simulink model "smlnk_hw3"  (R2019b)
settings: Solver=VariableStepAuto  StartTime=0.0  StopTime=30.0  RelTol=1e-3
undefined symbols (not defined in the file): K, k_r, L, ol, x0
settings Model: Creator=maximemeurisse  LastModifiedBy=maximemeurisse

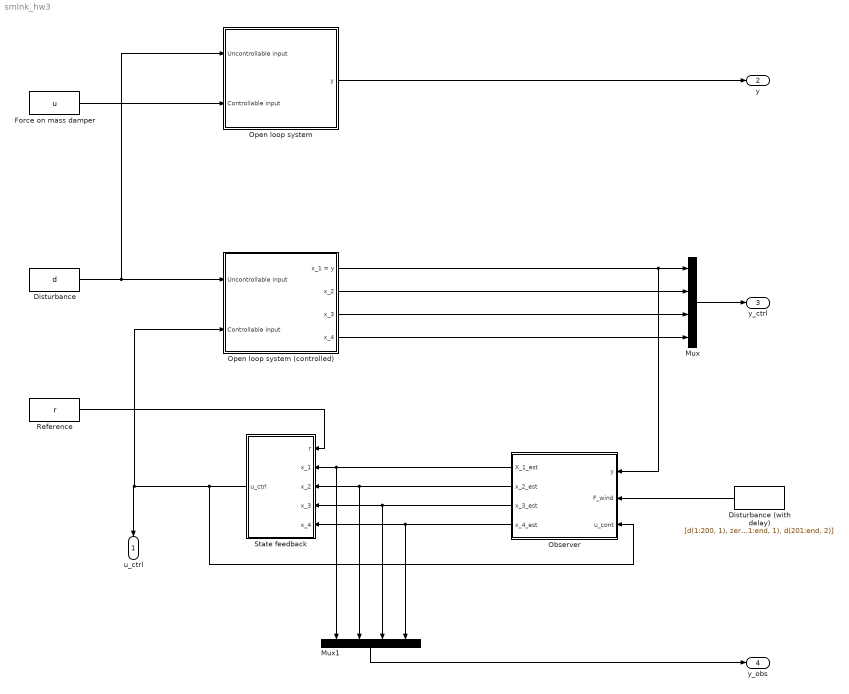
== system smlnk_hw3 ==
  Disturbance : FromWorkspace  VariableName=d  SampleTime=0
  Disturbance (with delay) : FromWorkspace  VariableName=[d(1:200, 1), zeros(200, 1); d(201:end, 1), d(201:end, 2)]  SampleTime=0
  Force on mass damper : FromWorkspace  VariableName=u  SampleTime=0
  Mux : Mux
  Mux1 : Mux
  Observer : Subsystem
  Open loop system : Subsystem
  Open loop system (controlled) : Subsystem
  Reference : FromWorkspace  VariableName=r  SampleTime=0
  State feedback : Subsystem
  u_ctrl : Outport
  y : Outport  Port=2
  y_ctrl : Outport  Port=3
  y_obs : Outport  Port=4
  wires:
  State feedback/1(u_ctrl) -> Observer/3(u_cont), Open loop system (controlled)/2(Controllable input), u_ctrl/1
  Observer/1(X_1_est) -> State feedback/2(x_1), Mux1/1
  Observer/2(x_2_est) -> State feedback/3(x_2), Mux1/2
  Reference/1 -> State feedback/1(r)
  Force on mass damper/1 -> Open loop system/2(Controllable input)
  Open loop system/1(y) -> y/1
  Mux/1 -> y_ctrl/1
  Mux1/1 -> y_obs/1
  Observer/3(x_3_est) -> State feedback/4(x_3), Mux1/3
  Observer/4(x_4_est) -> State feedback/5(x_4), Mux1/4
  Disturbance/1 -> Open loop system/1(Uncontrollable input), Open loop system (controlled)/1(Uncontrollable input)
  Open loop system (controlled)/2(x_2) -> Mux/2
  Open loop system (controlled)/3(x_3) -> Mux/3
  Open loop system (controlled)/4(x_4) -> Mux/4
  Open loop system (controlled)/1(x_1 = y) -> Observer/1(y), Mux/1
  Disturbance (with delay)/1 -> Observer/2(F_wind)

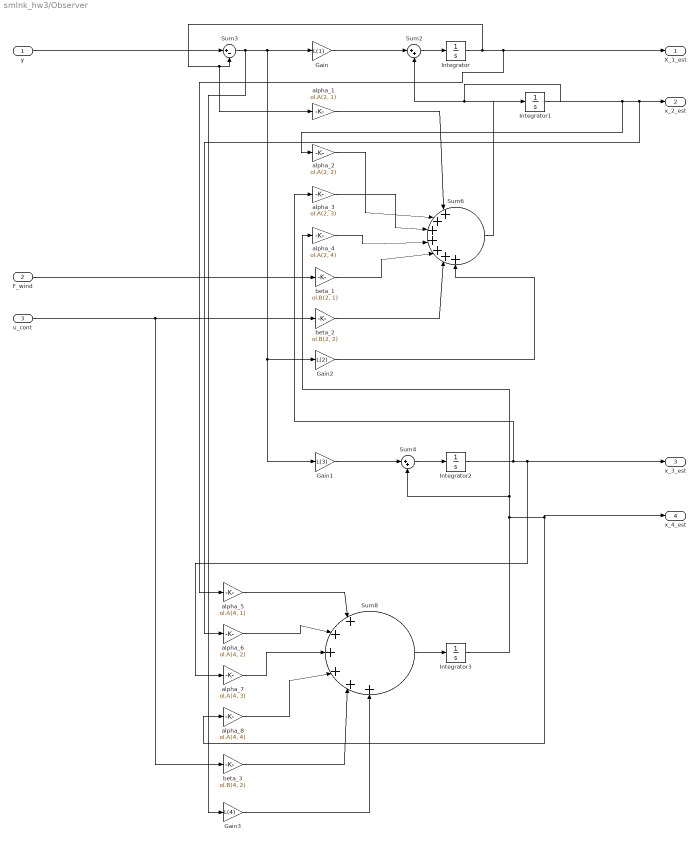
== system smlnk_hw3/Observer ==
  y : Inport
  F_wind : Inport  Port=2
  u_cont : Inport  Port=3
  Gain : Gain  Gain=L(1)
  Gain1 : Gain  Gain=L(3)
  Gain2 : Gain  Gain=L(2)
  Gain3 : Gain  Gain=L(4)
  Integrator{,1..3} (4 alike) : Integrator
  Sum2 : Sum  Inputs=|++
  Sum3 : Sum  Inputs=|+-
  Sum4 : Sum  Inputs=|++
  Sum6 : Sum  Inputs=|+++++++
  Sum8 : Sum  Inputs=|++++++
  alpha_1 : Gain  Gain=ol.A(2, 1)
  alpha_2 : Gain  Gain=ol.A(2, 2)
  alpha_3 : Gain  Gain=ol.A(2, 3)
  alpha_4 : Gain  Gain=ol.A(2, 4)
  alpha_5 : Gain  Gain=ol.A(4, 1)
  alpha_6 : Gain  Gain=ol.A(4, 2)
  alpha_7 : Gain  Gain=ol.A(4, 3)
  alpha_8 : Gain  Gain=ol.A(4, 4)
  beta_1 : Gain  Gain=ol.B(2, 1)
  beta_2 : Gain  Gain=ol.B(2, 2)
  beta_3 : Gain  Gain=ol.B(4, 2)
  X_1_est : Outport
  x_2_est : Outport  Port=2
  x_3_est : Outport  Port=3
  x_4_est : Outport  Port=4
  wires:
  Integrator2/1 -> alpha_3/1, alpha_7/1, x_3_est/1
  alpha_8/1 -> Sum8/4
  F_wind/1 -> beta_1/1
  Sum8/1 -> Integrator3/1
  alpha_2/1 -> Sum6/2
  beta_1/1 -> Sum6/5
  Sum4/1 -> Integrator2/1
  Integrator1/1 -> alpha_2/1, alpha_6/1, x_2_est/1, Sum2/2
  alpha_3/1 -> Sum6/3
  u_cont/1 -> beta_3/1, beta_2/1
  Gain1/1 -> Sum4/1
  alpha_4/1 -> Sum6/4
  Integrator/1 -> alpha_5/1, X_1_est/1, Sum3/2, alpha_1/1
  beta_3/1 -> Sum8/5
  Sum3/1 -> Gain3/1, Gain1/1, Gain2/1, Gain/1
  alpha_5/1 -> Sum8/1
  y/1 -> Sum3/1
  alpha_1/1 -> Sum6/1
  Sum2/1 -> Integrator/1
  alpha_6/1 -> Sum8/2
  beta_2/1 -> Sum6/6
  Sum6/1 -> Integrator1/1
  Gain2/1 -> Sum6/7
  Gain3/1 -> Sum8/6
  alpha_7/1 -> Sum8/3
  Gain/1 -> Sum2/1
  Integrator3/1 -> alpha_4/1, Sum4/2, alpha_8/1, x_4_est/1

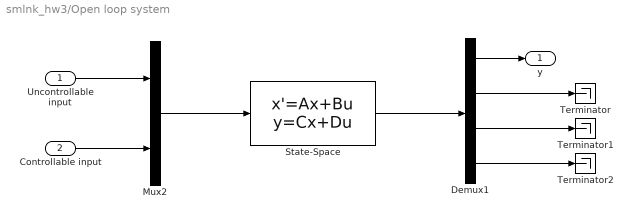
== system smlnk_hw3/Open loop system ==
  Uncontrollable input : Inport
  Controllable input : Inport  Port=2
  Demux1 : Demux
  Mux2 : Mux  Inputs=2
  State-Space : StateSpace  A=ol.A  B=ol.B  C=ol.C  D=ol.D  InitialCondition=x0
  Terminator : Terminator
  Terminator1 : Terminator
  Terminator2 : Terminator
  y : Outport
  wires:
  Controllable input/1 -> Mux2/2
  Uncontrollable input/1 -> Mux2/1
  Demux1/4 -> Terminator2/1
  Demux1/2 -> Terminator/1
  Demux1/3 -> Terminator1/1
  State-Space/1 -> Demux1/1
  Demux1/1 -> y/1
  Mux2/1 -> State-Space/1

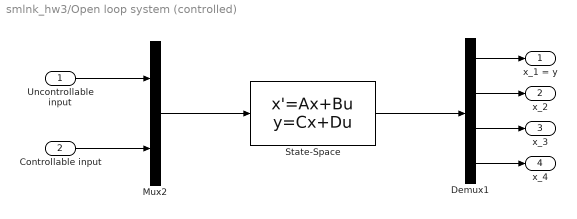
== system smlnk_hw3/Open loop system (controlled) ==
  Uncontrollable input : Inport
  Controllable input : Inport  Port=2
  Demux1 : Demux
  Mux2 : Mux  Inputs=2
  State-Space : StateSpace  A=ol.A  B=ol.B  C=ol.C  D=ol.D  InitialCondition=x0
  x_1 = y : Outport
  x_2 : Outport  Port=2
  x_3 : Outport  Port=3
  x_4 : Outport  Port=4
  wires:
  Controllable input/1 -> Mux2/2
  Uncontrollable input/1 -> Mux2/1
  Demux1/4 -> x_4/1
  Demux1/2 -> x_2/1
  Demux1/3 -> x_3/1
  State-Space/1 -> Demux1/1
  Demux1/1 -> x_1 = y/1
  Mux2/1 -> State-Space/1

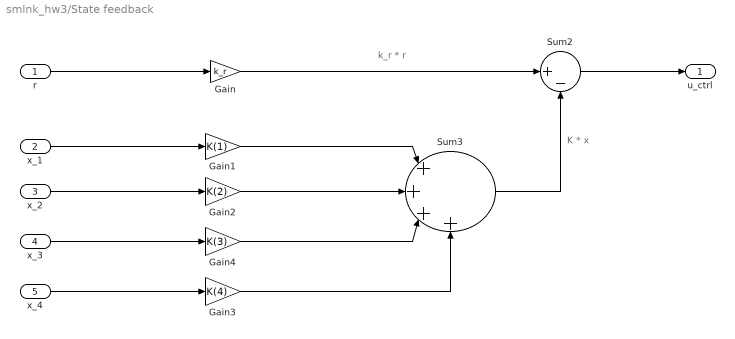
== system smlnk_hw3/State feedback ==
  note: K * x
  note: k_r * r
  r : Inport
  x_1 : Inport  Port=2
  x_2 : Inport  Port=3
  x_3 : Inport  Port=4
  x_4 : Inport  Port=5
  Gain : Gain  Gain=k_r
  Gain1 : Gain  Gain=K(1)
  Gain2 : Gain  Gain=K(2)
  Gain3 : Gain  Gain=K(4)
  Gain4 : Gain  Gain=K(3)
  Sum2 : Sum  Inputs=|+-
  Sum3 : Sum  Inputs=|++++
  u_ctrl : Outport
  wires:
  r/1 -> Gain/1
  x_4/1 -> Gain3/1
  x_1/1 -> Gain1/1
  Sum2/1 -> u_ctrl/1
  x_3/1 -> Gain4/1
  Sum3/1 -> Sum2/2
  Gain3/1 -> Sum3/4
  Gain/1 -> Sum2/1
  Gain1/1 -> Sum3/1
  x_2/1 -> Gain2/1
  Gain4/1 -> Sum3/3
  Gain2/1 -> Sum3/2
